simulink model "Pressure_DropPipeTheory_example"  (Simulink 7.6)
settings: Solver=ode45  StartTime=0.0  StopTime=10.0  RelTol=1e-3
libraries: carnot x2
settings Model: Creator=drhf  LastModifiedBy=drhf

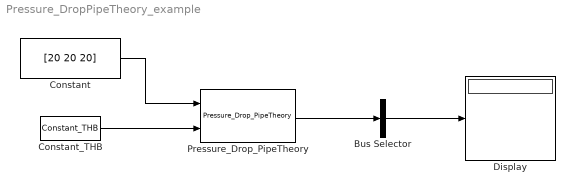
== system Pressure_DropPipeTheory_example ==
  Bus Selector : BusSelector  OutputSignals=Pressure,GeodeticHeight  OutputAsBus=on
  Constant : Constant  Value=[20 20 20]
  Constant_THB : carnot/Source/Simple/Constant_THB  SystemSampleTime=-1  t=40  mdot=200/3600  p=2e5  mID=Full Pressure Drop with Static Height  fluid=water  mix=0  dia=0.02  hgt=10
  Display : Display
  Pressure_Drop_PipeTheory : carnot/Basic/Pressure_Drop/Pressure_Drop_PipeTheory  SystemSampleTime=-1  dia=0.02  len=10  rough=0.04  nbend=1
  wires:
  Constant_THB/1 -> Pressure_Drop_PipeTheory/2
  Constant/1 -> Pressure_Drop_PipeTheory/1
  Pressure_Drop_PipeTheory/1 -> Bus Selector/1
  Bus Selector/1 -> Display/1
